simulink model "Final_Minh_Long"  (R2022b)
settings: Solver=VariableStepAuto  StartTime=0.0  StopTime=60  FixedStep=0.001  RelTol=1e-3
undefined symbols (not defined in the file): h, km, m, s, smiData, X, Y, Z
libraries: sm_lib x424, nesl_utility x32, aerolibconvert2 x25, simulink_extras x14, autolibshared x5, simulink x2
(part 1 of 11)
settings Model: Creator=dangm  LastModifiedBy=Lenovo
settings SolverCC: ZeroCrossAlgorithm=Adaptive  AlgebraicLoopSolver=LineSearch
settings DebuggingCC: IgnoredZcDiagnostic=none  UnconnectedInputMsg=warning  UnconnectedOutputMsg=warning  UnconnectedLineMsg=warning  SFMachineParentedDataDiag=warning
settings ModelReferenceCC: EnableRefExpFcnMdlSchedulingChecks=on

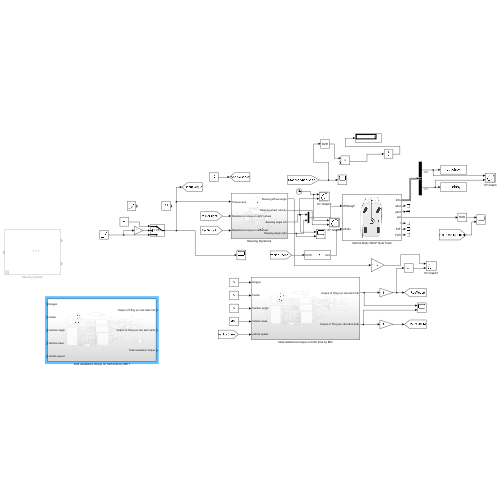
[thumbnail: Simulink's stored preview of the top-level diagram]
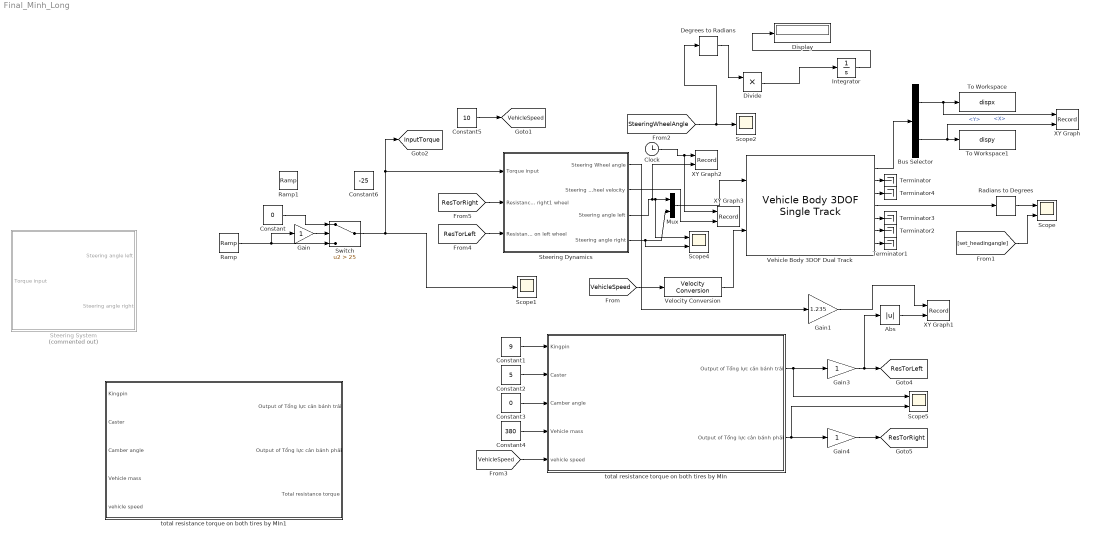
== system Final_Minh_Long ==
  Abs : Abs  SaturateOnIntegerOverflow=off
  Bus Selector : BusSelector  OutputSignals=InertFrm.Cg.Disp.X,InertFrm.Cg.Disp.Y
  Clock : Clock
  Constant : Constant  Value=0
  Constant1 : Constant  Value=9
  Constant2 : Constant  Value=5
  Constant3 : Constant  Value=0
  Constant4 : Constant  Value=380
  Constant5 : Constant  Value=10
  Constant6 : Constant  Value=-25
  Degrees to Radians : simulink_extras/Transformations/Degrees to Radians
  Display : Display
  Divide : Product  Inputs=**
  Gain : Gain
  Gain1 : Gain  Gain=1.235
  Gain3 : Gain
  Gain4 : Gain
  Integrator : Integrator
  Mux : Mux  Inputs=2
  Radians to Degrees : simulink_extras/Transformations/Radians to Degrees
  Ramp : simulink/Sources/Ramp  slope=1  start=0  InitialOutput=0
  Ramp1 : simulink/Sources/Ramp  slope=0.01  start=0  InitialOutput=0
  Scope : Scope  NumInputPorts=2
  Scope1 : Scope
  Scope2 : Scope
  Scope4 : Scope  NumInputPorts=2
  Scope5 : Scope  NumInputPorts=2
  Steering Dynamics : Subsystem
  Steering System : Subsystem  Commented=on
      mask Display: image('D:\MATLAB Projects\MATLAB_EPS_Complete_09_05\CapsoneProject\duy\mask\power-steering-2255498-1882000.png'); % Use "Edit Image" on toolstrip to change.
  Switch : Switch  Criteria=u2 > Threshold  Threshold=25  SaturateOnIntegerOverflow=off  InputSameDT=off
  Terminator{,1..4} (5 alike) : Terminator
  To Workspace : ToWorkspace  VariableName=dispx  SaveFormat=Structure With Time  SampleTime=-1
  To Workspace1 : ToWorkspace  VariableName=dispy  SaveFormat=Structure With Time  SampleTime=-1
  Vehicle Body 3DOF Dual Track : autolibshared/Vehicle Body 3DOF Single Track  trackMode=Dual  inputMode=External longitudinal velocity  frontSteerMode=on  rearSteerMode=off  windMode=off  muMode=off  extFMode=off  extMMode=off  htchFMode=off  htchMMode=off  extXo=off  extpsio=off  extxdoto=off  extro=off  extYo=off  extTamb=off  extydoto=off  aMode=2  NF=2  NR=2  m=1520  a=1.4  b=1.4  h=0.35  dh=1  hh=0.2  X_o=0  xdot_o=0  CalphaMode=off  sigmaMode=on  d=0  hl=0  w=[1.4,1.4]  Cy_f=12e3  Cy_r=11e3  sigma_f=.1  sigma_r=.1  alpha_f_brk=[-.1 .1]  Cy_f_data=[-9e3 9e3]  alpha_r_brk=[-.1 .1]  Cy_r_data=[-9e3 9e3]  Y_o=0  ydot_o=0  Izz=4000  psi_o=0  r_o=0  Af=2  Cd=.3  Cl=.1  Cpm=.1  beta_w=[0:0.01:0.3]  Cs=[0:0.03:0.9]  Cym=[0:0.01:0.3]  Pabs=101325  Tair=273  g=9.81  mu=1  xdot_tol=.01  Fznom=5000  Fxtire_sat=7e4  Fytire_sat=7e4  longOff=0  latOff=0  vertOff=0  wrapAng=off
  Velocity Conversion : aerolibconvert2/Velocity Conversion  IU=km/h  OU=m/s
  XY Graph : Record  FileSettingsInternal="{\"entries\":[{\"content\":{\"excelSettings\":{\"content\":{},\"type\":\"Streamout.ExcelSettings\"}},\"type\":\"Streamout.FileSettingStorage\",\"uuid\":\"20573330-48e2-4ccb-9357-96704c9ba468\"}],\"packageUris\":[\"http://schema.mathworks.com/mf0/streamout_blocks/R2020a\"],\"version\":\"1.0\"}"  Layout=[1 1]  SignalsInternal="{\"entries\":[{\"content\":{\"signals\":[{\"content\":{\"blockPath\":[\"Final_Minh_Long/XY Graph\"],\"channel\":[],\"dimensions\":[1],\"domain\":\"Final_Minh_Long/XY Graph\",\"lineColor\":\"#a2142f\",\"plots\":[1],\"port\":1,\"sid\":[\"\"],\"signalID\":3944,\"signalName\":\"<X>\"},\"type\":\"RecordBlkView.Signal\",\"uuid\":\"90b13e37-3913-4415-9f79-a5536db0b110\"},{\"content\":{\"blockPath\":[\"Final_Minh_Long/XY Graph\"],\"channel\":[],\"dimensions\":[1],\"domain\":\"Final_Minh_Long/XY Graph\",\"lineColor\":\"#139fff\",\"plots\":[1],\"port\":2,\"sid\":[\"\"],\"signalID\":3948,\"signalName\":\"<Y>\"},\"type\":\"RecordBlkView.Signal\",\"uuid\":\"8d3dad9d-9c13-4f6a-a484-58929b97bed7\"}]},\"type\":\"RecordBlkView.InputSignals\",\"uuid\":\"2abae3c5-8f03-4ddf-bdef-c417156e70b2\"}],\"packageUris\":[\"http://schema.mathworks.com/mf0/streamout_blocks/R2020a\"],\"version\":\"1.0\"}"  VisualizationBindings="{\"xyplotplugin\":{\"info\":[{\"series\":[{\"bindingParametersList\":[{\"parameter\":\"X-Axis\",\"signalID\":3944,\"signalName\":\"<X>\"},{\"parameter\":\"Y-Axis\",\"signalID\":3948,\"signalName\":\"<Y>\"}],\"seriesID\":57916}],\"subplotID\":1}]}}"  CompatibilityTag=XY  st=-1
  XY Graph1 : Record  FileSettingsInternal="{\"entries\":[{\"content\":{\"excelSettings\":{\"content\":{},\"type\":\"Streamout.ExcelSettings\"}},\"type\":\"Streamout.FileSettingStorage\",\"uuid\":\"0a007d86-071d-43f5-8a56-b751ea0b846e\"}],\"packageUris\":[\"http://schema.mathworks.com/mf0/streamout_blocks/R2020a\"],\"version\":\"1.0\"}"  Layout=[1 1]  SignalsInternal="{\"entries\":[{\"content\":{\"signals\":[{\"content\":{\"blockPath\":[\"Final_Minh_Long/XY Graph1\"],\"channel\":[],\"dimensions\":[1],\"domain\":\"Final_Minh_Long/XY Graph1\",\"lineColor\":\"#a2142f\",\"plots\":[1],\"port\":1,\"sid\":[\"\"],\"signalID\":3952,\"signalName\":\"Gain1\"},\"type\":\"RecordBlkView.Signal\",\"uuid\":\"8b19a18e-6e3d-497a-a0a3-2aad5dbcfb8c\"},{\"content\":{\"blockPath\":[\"Final_Minh_Long/XY Graph1\"],\"channel\":[],\"dimensions\":[1],\"domain\":\"Final_Minh_Long/XY Graph1\",\"lineColor\":\"#139fff\",\"plots\":[1],\"port\":2,\"sid\":[\"\"],\"signalID\":3956,\"signalName\":\"Abs\"},\"type\":\"RecordBlkView.Signal\",\"uuid\":\"0fb60146-9920-4be2-b459-6142f6fc3ce0\"}]},\"type\":\"RecordBlkView.InputSignals\",\"uuid\":\"4d27a010-d85b-49c4-9162-294f8bc1f08d\"}],\"packageUris\":[\"http://schema.mathworks.com/mf0/streamout_blocks/R2020a\"],\"version\":\"1.0\"}"  VisualizationBindings="{\"xyplotplugin\":{\"info\":[{\"series\":[{\"bindingParametersList\":[{\"parameter\":\"X-Axis\",\"signalID\":3952,\"signalName\":\"Gain1\"},{\"parameter\":\"Y-Axis\",\"signalID\":3956,\"signalName\":\"Abs\"}],\"seriesID\":31774}],\"subplotID\":1}]}}"  CompatibilityTag=XY  st=-1
  XY Graph2 : Record  FileSettingsInternal="{\"entries\":[{\"content\":{\"excelSettings\":{\"content\":{},\"type\":\"Streamout.ExcelSettings\"}},\"type\":\"Streamout.FileSettingStorage\",\"uuid\":\"818af3ad-4e78-4077-87d8-8a147781513b\"}],\"packageUris\":[\"http://schema.mathworks.com/mf0/streamout_blocks/R2020a\"],\"version\":\"1.0\"}"  Layout=[1 1]  SignalsInternal="{\"entries\":[{\"content\":{\"signals\":[{\"content\":{\"blockPath\":[\"Final_Minh_Long/XY Graph2\"],\"channel\":[],\"dimensions\":[1],\"domain\":\"Final_Minh_Long/XY Graph2\",\"lineColor\":\"#a2142f\",\"plots\":[1],\"port\":1,\"sid\":[\"\"],\"signalID\":3960,\"signalName\":\"Clock\"},\"type\":\"RecordBlkView.Signal\",\"uuid\":\"f2a8c6ab-ef34-4918-a704-d61b8c315ada\"},{\"content\":{\"blockPath\":[\"Final_Minh_Long/XY Graph2\"],\"channel\":[],\"dimensions\":[1],\"domain\":\"Final_Minh_Long/XY Graph2\",\"lineColor\":\"#139fff\",\"plots\":[1],\"port\":2,\"sid\":[\"\"],\"signalID\":3964,\"signalName\":\"Steering Dynamics:3\"},\"type\":\"RecordBlkView.Signal\",\"uuid\":\"651528bd-dcb0-49c9-af94-924e8d19c524\"}]},\"type\":\"RecordBlkView.InputSignals\",\"uuid\":\"f8b33b09-6380-4f4b-ae2b-7c84b78898a2\"}],\"packageUris\":[\"http://schema.mathworks.com/mf0/streamout_blocks/R2020a\"],\"version\":\"1.0\"}"  VisualizationBindings="{\"xyplotplugin\":{\"info\":[{\"series\":[{\"bindingParametersList\":[{\"parameter\":\"X-Axis\",\"signalID\":3960,\"signalName\":\"Clock\"},{\"parameter\":\"Y-Axis\",\"signalID\":3964,\"signalName\":\"Steering Dynamics:3\"}],\"seriesID\":31371}],\"subplotID\":1}]}}"  CompatibilityTag=XY  st=-1
  XY Graph3 : Record  FileSettingsInternal="{\"entries\":[{\"content\":{\"excelSettings\":{\"content\":{},\"type\":\"Streamout.ExcelSettings\"}},\"type\":\"Streamout.FileSettingStorage\",\"uuid\":\"88566568-d1b9-45b3-b9ae-773698c52360\"}],\"packageUris\":[\"http://schema.mathworks.com/mf0/streamout_blocks/R2020a\"],\"version\":\"1.0\"}"  Layout=[1 1]  SignalsInternal="{\"entries\":[{\"content\":{\"signals\":[{\"content\":{\"blockPath\":[\"Final_Minh_Long/XY Graph3\"],\"channel\":[],\"dimensions\":[1],\"domain\":\"Final_Minh_Long/XY Graph3\",\"lineColor\":\"#a2142f\",\"plots\":[1],\"port\":1,\"sid\":[\"\"],\"signalID\":3968,\"signalName\":\"Clock\"},\"type\":\"RecordBlkView.Signal\",\"uuid\":\"cc2650eb-84e2-4086-96a6-97ce3e4d41ed\"},{\"content\":{\"blockPath\":[\"Final_Minh_Long/XY Graph3\"],\"channel\":[],\"dimensions\":[1],\"domain\":\"Final_Minh_Long/XY Graph3\",\"lineColor\":\"#139fff\",\"plots\":[1],\"port\":2,\"sid\":[\"\"],\"signalID\":3972,\"signalName\":\"Steering Dynamics:2\"},\"type\":\"RecordBlkView.Signal\",\"uuid\":\"bed2728c-8836-43cf-9a2f-cf65613dc0e0\"}]},\"type\":\"RecordBlkView.InputSignals\",\"uuid\":\"f26de753-25e0-4fe3-9a2b-f6db05d15f66\"}],\"packageUris\":[\"http://schema.mathworks.com/mf0/streamout_blocks/R2020a\"],\"version\":\"1.0\"}"  VisualizationBindings="{\"xyplotplugin\":{\"info\":[{\"series\":[{\"bindingParametersList\":[{\"parameter\":\"X-Axis\",\"signalID\":3968,\"signalName\":\"Clock\"},{\"parameter\":\"Y-Axis\",\"signalID\":3972,\"signalName\":\"Steering Dynamics:2\"}],\"seriesID\":17655}],\"subplotID\":1}]}}"  CompatibilityTag=XY  st=-1
  total resistance torque on both tires by MIn : Subsystem
  total resistance torque on both tires by MIn1 : Subsystem
  tag scope: InputTorque=global, ResTorLeft=global, ResTorRight=global, VehicleSpeed=global
  wires:
  Mux/1 -> Vehicle Body 3DOF Dual Track/1
  Vehicle Body 3DOF Dual Track/7 -> Terminator1/1
  Vehicle Body 3DOF Dual Track/6 -> Terminator2/1
  Vehicle Body 3DOF Dual Track/5 -> Terminator3/1
  Vehicle Body 3DOF Dual Track/1 -> Bus Selector/1
  Bus Selector/1 -> XY Graph/1, To Workspace/1  "<X>"
  Bus Selector/2 -> XY Graph/2, To Workspace1/1  "<Y>"
  Velocity Conversion/1 -> Vehicle Body 3DOF Dual Track/2
  [VehicleSpeed] -> Velocity Conversion/1
  Constant5/1 -> [VehicleSpeed]
  Vehicle Body 3DOF Dual Track/2 -> Terminator/1
  Vehicle Body 3DOF Dual Track/3 -> Terminator4/1
  Vehicle Body 3DOF Dual Track/4 -> Radians to Degrees/1
  Radians to Degrees/1 -> Scope/1
  [set_headingangle] -> Scope/2
  [SteeringWheelAngle] -> Scope2/1, Degrees to Radians/1
  Gain4/1 -> [ResTorRight]
  Gain3/1 -> Abs/1, [ResTorLeft]
  Constant1/1 -> total resistance torque on both tires by MIn/1(Kingpin)
  Constant4/1 -> total resistance torque on both tires by MIn/4(Vehicle mass)
  Constant3/1 -> total resistance torque on both tires by MIn/3(Camber angle)
  Constant2/1 -> total resistance torque on both tires by MIn/2(Caster)
  total resistance torque on both tires by MIn/1(Output of Tổng lực cản bánh trái) -> Scope5/1, Gain3/1
  total resistance torque on both tires by MIn/2(Output of Tổng lực cản bánh phải) -> Gain4/1, Scope5/2
  [VehicleSpeed] -> total resistance torque on both tires by MIn/5("vehicle speed ")
  Degrees to Radians/1 -> Divide/1
  Divide/1 -> Integrator/1
  Integrator/1 -> Display/1
  Constant/1 -> Switch/1
  Switch/1 -> Scope1/1, [InputTorque], Steering Dynamics/1(Torque input)
  Ramp/1 -> Gain/1, Switch/3
  Steering Dynamics/3(Steering angle left) -> XY Graph2/2, Scope4/1, Mux/1
  Steering Dynamics/4(Steering angle right) -> Scope4/2, Mux/2
  [ResTorRight] -> Steering Dynamics/2(Resistance torque on right1 wheel)
  [ResTorLeft] -> Steering Dynamics/3(Resistance torque on left wheel)
  Steering Dynamics/1(Steering Wheel angle) -> Gain1/1
  Gain/1 -> Switch/2
  Abs/1 -> XY Graph1/2
  Gain1/1 -> XY Graph1/1
  Clock/1 -> XY Graph3/1, XY Graph2/1
  Steering Dynamics/2(Steering wheel velocity) -> XY Graph3/2

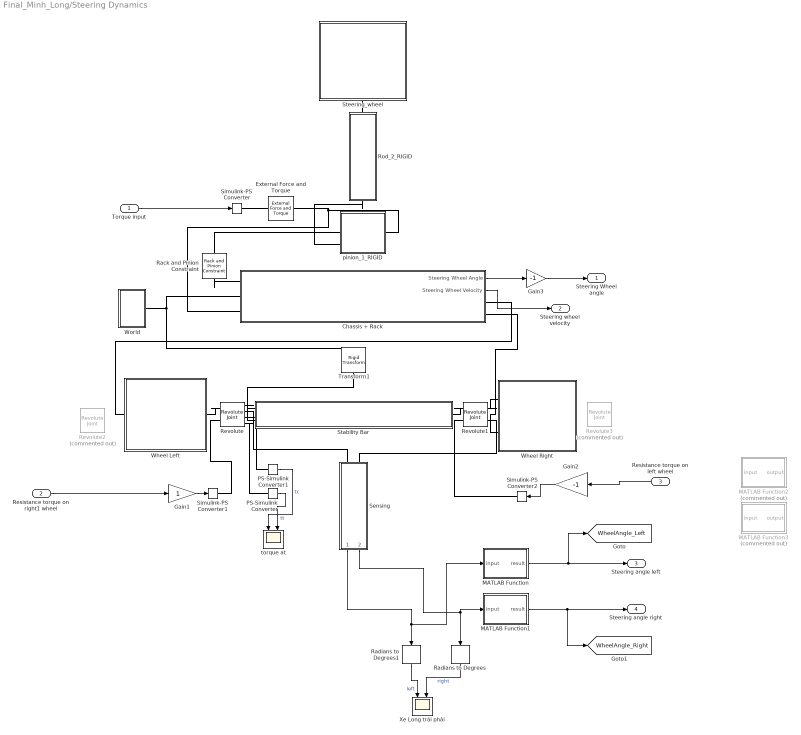
== system Final_Minh_Long/Steering Dynamics ==
  Torque input : Inport
  Resistance torque on right1 wheel : Inport  Port=2
  Resistance torque on left wheel : Inport  Port=3
  Chassis + Rack : Subsystem
      mask Display: image('$imagefile'); % Use "Edit Image" on toolstrip to change.
  External Force and Torque : sm_lib/Forces and Torques/External Force and Torque  ForceResolutionFrame=AttachedFrame  EnableForceX=off  EnableForceY=off  EnableForceZ=off  EnableForce=off  TorqueResolutionFrame=AttachedFrame  EnableTorqueX=off  EnableTorqueY=off  EnableTorqueZ=on  EnableTorque=off
  Gain1 : Gain
  Gain2 : Gain  Gain=-1
  Gain3 : Gain  Gain=-1
  MATLAB Function : MATLAB Function  TreatAsAtomicUnit=on
  MATLAB Function1 : MATLAB Function  TreatAsAtomicUnit=on
  MATLAB Function2 : MATLAB Function  Commented=on  TreatAsAtomicUnit=on
  MATLAB Function3 : MATLAB Function  Commented=on  TreatAsAtomicUnit=on
  PS-Simulink Converter : nesl_utility/PS-Simulink Converter  PhysicalDomain=network_engine_domain  SubClassName=ps_output  LeftPortType=input  RightPortType=output  PseudoPeriodic=off  Frequencies=[]  VectorFormat=1-D array  Unit=inherit  AffineConversion=off
  PS-Simulink Converter1 : nesl_utility/PS-Simulink Converter  PhysicalDomain=network_engine_domain  SubClassName=ps_output  LeftPortType=input  RightPortType=output  PseudoPeriodic=off  Frequencies=[]  VectorFormat=1-D array  Unit=inherit  AffineConversion=off
  Rack and Pinion Constraint : sm_lib/Gears and Couplings/Gears/Rack and Pinion Constraint  PinionRadius=30  PinionRadiusUnits=mm
  Radians to Degrees : simulink_extras/Transformations/Radians to Degrees
  Radians to Degrees1 : simulink_extras/Transformations/Radians to Degrees
  Revolute : sm_lib/Joints/Revolute Joint  JointMode=Normal  SenseConstraintForce=off  SenseConstraintForceX=off  SenseConstraintForceY=off  SenseConstraintForceZ=off  SenseConstraintTorque=on  SenseConstraintTorqueX=off  SenseConstraintTorqueY=off  SenseConstraintTorqueZ=off  SenseTotalForce=off  SenseTotalForceX=off  SenseTotalForceY=off  SenseTotalForceZ=off  SenseTotalTorque=on  SenseTotalTorqueX=off  SenseTotalTorqueY=off  SenseTotalTorqueZ=off  CompositeWrenchDir=BaseOnFollower  CompositeWrenchFrame=FollowerFrame  EquilibriumPosition=0  EquilibriumPositionUnits=deg  SpringStiffness=0.0524-0.0524  SpringStiffnessUnits=N*m/deg  DampingCoefficient=1.5-1.5+0.1  DampingCoefficientUnits=N*m/(deg/s)  TorqueActuationMode=InputTorque  MotionActuationMode=ComputedMotion  SensePosition=on  SenseVelocity=off  SenseAcceleration=off  SenseTorqueForce=off  SenseLowerLimitTorqueForce=off  SenseUpperLimitTorqueForce=off  LowerLimitSpecify=on  LowerLimitBound=-89.68-28.95  LowerLimitBoundUnits=deg  LowerLimitStiffness=1e4  LowerLimitStiffnessUnits=N*m/deg  LowerLimitDamping=100  LowerLimitDampingUnits=N*m/(deg/s)  LowerLimitTransitionRegionWidth=0.1  LowerLimitTransitionRegionWidthUnits=deg  UpperLimitSpecify=on  UpperLimitBound=-89.68+18.80  UpperLimitBoundUnits=deg  UpperLimitStiffness=1e4  UpperLimitStiffnessUnits=N*m/deg  UpperLimitDamping=100  UpperLimitDampingUnits=N*m/(deg/s)  UpperLimitTransitionRegionWidth=0.1  UpperLimitTransitionRegionWidthUnits=deg  PositionTargetSpecify=on  PositionTargetPriority=High  PositionTargetValue=-89.678329494  PositionTargetValueUnits=deg  VelocityTargetSpecify=on  VelocityTargetPriority=High  VelocityTargetValue=0  VelocityTargetValueUnits=deg/s
  Revolute1 : sm_lib/Joints/Revolute Joint  JointMode=Normal  SenseConstraintForce=off  SenseConstraintForceX=off  SenseConstraintForceY=off  SenseConstraintForceZ=off  SenseConstraintTorque=off  SenseConstraintTorqueX=off  SenseConstraintTorqueY=off  SenseConstraintTorqueZ=off  SenseTotalForce=off  SenseTotalForceX=off  SenseTotalForceY=off  SenseTotalForceZ=off  SenseTotalTorque=off  SenseTotalTorqueX=off  SenseTotalTorqueY=off  SenseTotalTorqueZ=off  CompositeWrenchDir=FollowerOnBase  CompositeWrenchFrame=FollowerFrame  EquilibriumPosition=0  EquilibriumPositionUnits=deg  SpringStiffness=0  SpringStiffnessUnits=N*m/deg  DampingCoefficient=0.1  DampingCoefficientUnits=N*m/(deg/s)  TorqueActuationMode=InputTorque  MotionActuationMode=ComputedMotion  SensePosition=on  SenseVelocity=off  SenseAcceleration=off  SenseTorqueForce=off  SenseLowerLimitTorqueForce=off  SenseUpperLimitTorqueForce=off  LowerLimitSpecify=on  LowerLimitBound=-89.68-28.95  LowerLimitBoundUnits=deg  LowerLimitStiffness=1e4  LowerLimitStiffnessUnits=N*m/deg  LowerLimitDamping=100  LowerLimitDampingUnits=N*m/(deg/s)  LowerLimitTransitionRegionWidth=0.1  LowerLimitTransitionRegionWidthUnits=deg  UpperLimitSpecify=on  UpperLimitBound=-89.68+18.80  UpperLimitBoundUnits=deg  UpperLimitStiffness=1e4  UpperLimitStiffnessUnits=N*m/deg  UpperLimitDamping=100  UpperLimitDampingUnits=N*m/(deg/s)  UpperLimitTransitionRegionWidth=0.1  UpperLimitTransitionRegionWidthUnits=deg  PositionTargetSpecify=on  PositionTargetPriority=Low  PositionTargetValue=smiData.RevoluteJoint(2).Rz.Pos-2.7  PositionTargetValueUnits=deg  VelocityTargetSpecify=on  VelocityTargetPriority=High  VelocityTargetValue=0  VelocityTargetValueUnits=deg/s
  Revolute2 : sm_lib/Joints/Revolute Joint  Commented=on  JointMode=Normal  SenseConstraintForce=off  SenseConstraintForceX=off  SenseConstraintForceY=off  SenseConstraintForceZ=off  SenseConstraintTorque=off  SenseConstraintTorqueX=off  SenseConstraintTorqueY=off  SenseConstraintTorqueZ=off  SenseTotalForce=off  SenseTotalForceX=off  SenseTotalForceY=off  SenseTotalForceZ=off  SenseTotalTorque=off  SenseTotalTorqueX=off  SenseTotalTorqueY=off  SenseTotalTorqueZ=off  CompositeWrenchDir=BaseOnFollower  CompositeWrenchFrame=FollowerFrame  EquilibriumPosition=0  EquilibriumPositionUnits=deg  SpringStiffness=0.0524-0.0524+0.1  SpringStiffnessUnits=N*m/deg  DampingCoefficient=1.5-1.5+0.1  DampingCoefficientUnits=N*m/(deg/s)  TorqueActuationMode=InputTorque  MotionActuationMode=ComputedMotion  SensePosition=on  SenseVelocity=off  SenseAcceleration=off  SenseTorqueForce=off  SenseLowerLimitTorqueForce=off  SenseUpperLimitTorqueForce=off  LowerLimitSpecify=on  LowerLimitBound=-2+0.089+0.071  LowerLimitBoundUnits=rad  LowerLimitStiffness=1e4  LowerLimitStiffnessUnits=N*m/deg  LowerLimitDamping=100  LowerLimitDampingUnits=N*m/(deg/s)  LowerLimitTransitionRegionWidth=0.1  LowerLimitTransitionRegionWidthUnits=deg  UpperLimitSpecify=on  UpperLimitBound=-1-0.195-0.106  UpperLimitBoundUnits=rad  UpperLimitStiffness=1e4  UpperLimitStiffnessUnits=N*m/deg  UpperLimitDamping=100  UpperLimitDampingUnits=N*m/(deg/s)  UpperLimitTransitionRegionWidth=0.1  UpperLimitTransitionRegionWidthUnits=deg  PositionTargetSpecify=on  PositionTargetPriority=High  PositionTargetValue=-89.678329494  PositionTargetValueUnits=deg  VelocityTargetSpecify=on  VelocityTargetPriority=High  VelocityTargetValue=0  VelocityTargetValueUnits=deg/s
  Revolute3 : sm_lib/Joints/Revolute Joint  Commented=on  JointMode=Normal  SenseConstraintForce=off  SenseConstraintForceX=off  SenseConstraintForceY=off  SenseConstraintForceZ=off  SenseConstraintTorque=off  SenseConstraintTorqueX=off  SenseConstraintTorqueY=off  SenseConstraintTorqueZ=off  SenseTotalForce=off  SenseTotalForceX=off  SenseTotalForceY=off  SenseTotalForceZ=off  SenseTotalTorque=off  SenseTotalTorqueX=off  SenseTotalTorqueY=off  SenseTotalTorqueZ=off  CompositeWrenchDir=FollowerOnBase  CompositeWrenchFrame=FollowerFrame  EquilibriumPosition=0  EquilibriumPositionUnits=deg  SpringStiffness=0.1  SpringStiffnessUnits=N*m/deg  DampingCoefficient=0.1  DampingCoefficientUnits=N*m/(deg/s)  TorqueActuationMode=InputTorque  MotionActuationMode=ComputedMotion  SensePosition=on  SenseVelocity=off  SenseAcceleration=off  SenseTorqueForce=off  SenseLowerLimitTorqueForce=off  SenseUpperLimitTorqueForce=off  LowerLimitSpecify=off  LowerLimitBound=-2  LowerLimitBoundUnits=rad  LowerLimitStiffness=1e4  LowerLimitStiffnessUnits=N*m/deg  LowerLimitDamping=100  LowerLimitDampingUnits=N*m/(deg/s)  LowerLimitTransitionRegionWidth=0.1  LowerLimitTransitionRegionWidthUnits=deg  UpperLimitSpecify=off  UpperLimitBound=-1  UpperLimitBoundUnits=rad  UpperLimitStiffness=1e4  UpperLimitStiffnessUnits=N*m/deg  UpperLimitDamping=100  UpperLimitDampingUnits=N*m/(deg/s)  UpperLimitTransitionRegionWidth=0.1  UpperLimitTransitionRegionWidthUnits=deg  PositionTargetSpecify=on  PositionTargetPriority=Low  PositionTargetValue=smiData.RevoluteJoint(2).Rz.Pos-2.7  PositionTargetValueUnits=deg  VelocityTargetSpecify=on  VelocityTargetPriority=High  VelocityTargetValue=0  VelocityTargetValueUnits=deg/s
  Rod_2_RIGID : Subsystem
      mask Display: image('rod.png'); % Use "Edit Image" on toolstrip to change.
  "Sensing " : Subsystem
  Simulink-PS Converter : nesl_utility/Simulink-PS Converter  PhysicalDomain=network_engine_domain  SubClassName=ps_input  LeftPortType=input  RightPortType=output  PseudoPeriodic=off  Frequencies=[]  NoiseDistribution=none  NoiseParameters=[]  Unit=N*m  AffineConversion=off  FilteringAndDerivatives=provide  SimscapeFilterOrder=1  InputFilterTimeConstant=0.001  UdotUserProvided=0
  Simulink-PS Converter1 : nesl_utility/Simulink-PS Converter  PhysicalDomain=network_engine_domain  SubClassName=ps_input  LeftPortType=input  RightPortType=output  PseudoPeriodic=off  Frequencies=[]  NoiseDistribution=none  NoiseParameters=[]  Unit=N*m  AffineConversion=off  FilteringAndDerivatives=provide  SimscapeFilterOrder=1  InputFilterTimeConstant=0.001  UdotUserProvided=0
  Simulink-PS Converter2 : nesl_utility/Simulink-PS Converter  PhysicalDomain=network_engine_domain  SubClassName=ps_input  LeftPortType=input  RightPortType=output  PseudoPeriodic=off  Frequencies=[]  NoiseDistribution=none  NoiseParameters=[]  Unit=N*m  AffineConversion=off  FilteringAndDerivatives=provide  SimscapeFilterOrder=2  InputFilterTimeConstant=0.001  UdotUserProvided=0
  Stability Bar : Subsystem
      mask Display: image('$imagefile'); % Use "Edit Image" on toolstrip to change.
  Steering_wheel : Subsystem
      mask Display: image('$imagefile'); % Use "Edit Image" on toolstrip to change.
  Transform1 : sm_lib/Frames and Transforms/Rigid Transform  TranslationMethod=Cartesian  TranslationStandardOffset=0  TranslationLengthUnit=mm  TranslationStandardAxis=+Z  TranslationCartesianOffset=smiData.RigidTransform(48).translation  TranslationROffset=0  TranslationROffsetUnits=m  TranslationZOffset=0  TranslationZOffsetUnits=m  TranslationThetaOffset=0  TranslationThetaOffsetUnits=deg  RotationMethod=ArbitraryAxis  RotationAngleUnits=rad  RotationStandardAxis=+Z  RotationAngle=smiData.RigidTransform(48).angle  RotationArbitraryAxis=smiData.RigidTransform(48).axis  FollAlignAxisA=+X  BaseAlignAxisA=+Y  FollAlignAxisB=+Y  BaseAlignAxisB=+Z  RotationSequenceAxes=FollowerAxes  RotationSequence=XYX  RotationSequenceAngles=[0 0 0]  RotationSequenceAnglesUnits=deg  RotationMatrix=[1 0 0; 0 1 0; 0 0 1]  Quaternion=[1 0 0 0]
  Wheel Left : Subsystem
      mask Display: image('$imagefile'); % Use "Edit Image" on toolstrip to change.
  Wheel Right : Subsystem
      mask Display: image('$imagefile'); % Use "Edit Image" on toolstrip to change.
  World : Subsystem
  Xe Long trái phải : Scope  NumInputPorts=2
  pinion_1_RIGID : Subsystem
      mask Display: image('pinion.png'); % Use "Edit Image" on toolstrip to change.
  "torque at " : Scope  NumInputPorts=2
  Steering Wheel angle : Outport
  Steering wheel velocity : Outport  Port=2
  Steering angle left : Outport  Port=3
  Steering angle right : Outport  Port=4
  tag scope: WheelAngle_Left=global, WheelAngle_Right=global
  wires:
  "Sensing "/2(Steering angle right (rad)) -> MATLAB Function1/1(input), Radians to Degrees/1
  Radians to Degrees/1 -> Xe Long trái phải/2  "right"
  Radians to Degrees1/1 -> Xe Long trái phải/1  "left"
  Chassis + Rack/2(Steering Wheel Velocity) -> Steering wheel velocity/1
  Chassis + Rack/1(Steering Wheel Angle) -> Gain3/1
  Resistance torque on right1 wheel/1 -> Gain1/1
  Resistance torque on left wheel/1 -> Gain2/1
  Gain1/1 -> Simulink-PS Converter1/1
  Gain2/1 -> Simulink-PS Converter2/1
  MATLAB Function/1(result) -> [WheelAngle_Left], Steering angle left/1
  MATLAB Function1/1(result) -> [WheelAngle_Right], Steering angle right/1
  "Sensing "/1(Steering angle left (rad)) -> Radians to Degrees1/1, MATLAB Function/1(input)
  PS-Simulink Converter1/1 -> "torque at "/1  "tc"
  PS-Simulink Converter/1 -> "torque at "/2  "tt"
  Torque input/1 -> Simulink-PS Converter/1
  Gain3/1 -> Steering Wheel angle/1
  connections:
  Revolute/RConn2 -- "Sensing "/LConn1
  Simulink-PS Converter/RConn1 -- External Force and Torque/LConn1
  Chassis + Rack/LConn2 -- World/LConn1 -- Transform1/LConn1
  Rack and Pinion Constraint/RConn1 -- Chassis + Rack/LConn1
  Revolute1/RConn2 -- "Sensing "/LConn2
  Rack and Pinion Constraint/LConn1 -- pinion_1_RIGID/LConn2
  Transform1/RConn1 -- Stability Bar/LConn2
  Chassis + Rack/LConn3 -- pinion_1_RIGID/RConn1 -- External Force and Torque/RConn1
  Chassis + Rack/RConn1 -- Wheel Left/LConn1
  Revolute1/RConn1 -- Wheel Right/LConn1
  Chassis + Rack/RConn2 -- Wheel Right/LConn2
  Revolute1/LConn1 -- Stability Bar/RConn1
  Revolute/RConn1 -- Stability Bar/LConn1
  Revolute/LConn1 -- Wheel Left/RConn1
  Rod_2_RIGID/RConn1 -- pinion_1_RIGID/LConn3
  Steering_wheel/LConn1 -- Rod_2_RIGID/LConn1
  Simulink-PS Converter1/RConn1 -- Revolute/LConn2
  Revolute1/LConn2 -- Simulink-PS Converter2/RConn1
  Revolute/RConn3 -- PS-Simulink Converter1/LConn1
  Revolute/RConn4 -- PS-Simulink Converter/LConn1

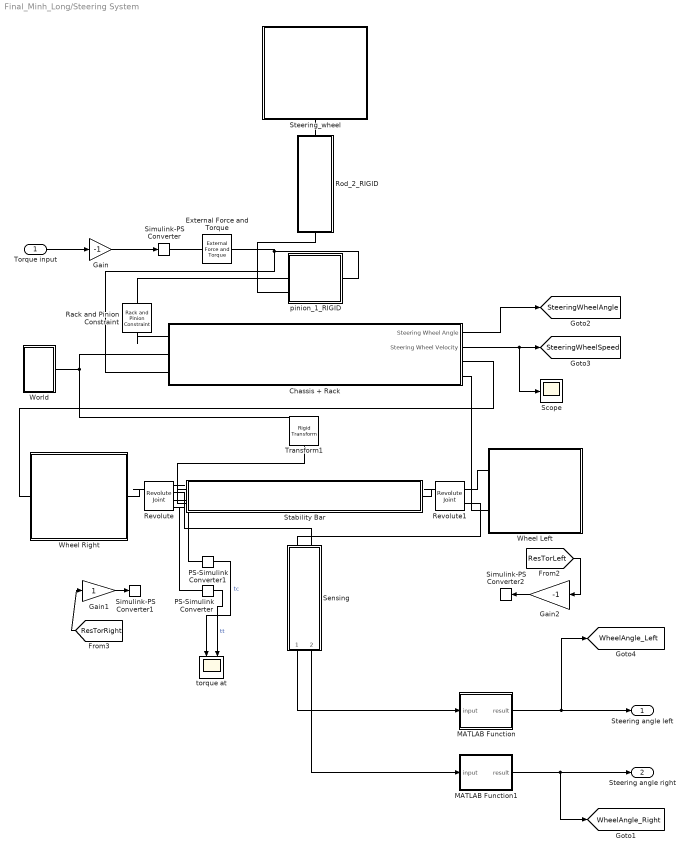
== system Final_Minh_Long/Steering System ==
  Torque input : Inport
  Chassis + Rack : Subsystem
      mask Display: image('$imagefile'); % Use "Edit Image" on toolstrip to change.
  External Force and Torque : sm_lib/Forces and Torques/External Force and Torque  ForceResolutionFrame=AttachedFrame  EnableForceX=off  EnableForceY=off  EnableForceZ=off  EnableForce=off  TorqueResolutionFrame=AttachedFrame  EnableTorqueX=off  EnableTorqueY=off  EnableTorqueZ=on  EnableTorque=off
  Gain : Gain  Gain=-1
  Gain1 : Gain
  Gain2 : Gain  Gain=-1
  MATLAB Function : MATLAB Function  TreatAsAtomicUnit=on
  MATLAB Function1 : MATLAB Function  TreatAsAtomicUnit=on
  PS-Simulink Converter : nesl_utility/PS-Simulink Converter  PhysicalDomain=network_engine_domain  SubClassName=ps_output  LeftPortType=input  RightPortType=output  PseudoPeriodic=off  Frequencies=[]  VectorFormat=1-D array  Unit=inherit  AffineConversion=off
  PS-Simulink Converter1 : nesl_utility/PS-Simulink Converter  PhysicalDomain=network_engine_domain  SubClassName=ps_output  LeftPortType=input  RightPortType=output  PseudoPeriodic=off  Frequencies=[]  VectorFormat=1-D array  Unit=inherit  AffineConversion=off
  Rack and Pinion Constraint : sm_lib/Gears and Couplings/Gears/Rack and Pinion Constraint  PinionRadius=30  PinionRadiusUnits=mm
  Revolute : sm_lib/Joints/Revolute Joint  JointMode=Normal  SenseConstraintForce=off  SenseConstraintForceX=off  SenseConstraintForceY=off  SenseConstraintForceZ=off  SenseConstraintTorque=on  SenseConstraintTorqueX=off  SenseConstraintTorqueY=off  SenseConstraintTorqueZ=off  SenseTotalForce=off  SenseTotalForceX=off  SenseTotalForceY=off  SenseTotalForceZ=off  SenseTotalTorque=on  SenseTotalTorqueX=off  SenseTotalTorqueY=off  SenseTotalTorqueZ=off  CompositeWrenchDir=BaseOnFollower  CompositeWrenchFrame=FollowerFrame  EquilibriumPosition=0  EquilibriumPositionUnits=deg  SpringStiffness=0.0524-0.0524+0.1  SpringStiffnessUnits=N*m/deg  DampingCoefficient=1.5-1.5+0.1  DampingCoefficientUnits=N*m/(deg/s)  TorqueActuationMode=InputTorque  MotionActuationMode=ComputedMotion  SensePosition=on  SenseVelocity=off  SenseAcceleration=off  SenseTorqueForce=off  SenseLowerLimitTorqueForce=off  SenseUpperLimitTorqueForce=off  LowerLimitSpecify=on  LowerLimitBound=-89.68-28.95  LowerLimitBoundUnits=deg  LowerLimitStiffness=1e4  LowerLimitStiffnessUnits=N*m/deg  LowerLimitDamping=100  LowerLimitDampingUnits=N*m/(deg/s)  LowerLimitTransitionRegionWidth=0.1  LowerLimitTransitionRegionWidthUnits=deg  UpperLimitSpecify=on  UpperLimitBound=-89.68+18.80  UpperLimitBoundUnits=deg  UpperLimitStiffness=1e4  UpperLimitStiffnessUnits=N*m/deg  UpperLimitDamping=100  UpperLimitDampingUnits=N*m/(deg/s)  UpperLimitTransitionRegionWidth=0.1  UpperLimitTransitionRegionWidthUnits=deg  PositionTargetSpecify=on  PositionTargetPriority=High  PositionTargetValue=-89.678329494  PositionTargetValueUnits=deg  VelocityTargetSpecify=on  VelocityTargetPriority=High  VelocityTargetValue=0  VelocityTargetValueUnits=deg/s
  Revolute1 : sm_lib/Joints/Revolute Joint  JointMode=Normal  SenseConstraintForce=off  SenseConstraintForceX=off  SenseConstraintForceY=off  SenseConstraintForceZ=off  SenseConstraintTorque=off  SenseConstraintTorqueX=off  SenseConstraintTorqueY=off  SenseConstraintTorqueZ=off  SenseTotalForce=off  SenseTotalForceX=off  SenseTotalForceY=off  SenseTotalForceZ=off  SenseTotalTorque=off  SenseTotalTorqueX=off  SenseTotalTorqueY=off  SenseTotalTorqueZ=off  CompositeWrenchDir=FollowerOnBase  CompositeWrenchFrame=FollowerFrame  EquilibriumPosition=0  EquilibriumPositionUnits=deg  SpringStiffness=0.1  SpringStiffnessUnits=N*m/deg  DampingCoefficient=0.1  DampingCoefficientUnits=N*m/(deg/s)  TorqueActuationMode=InputTorque  MotionActuationMode=ComputedMotion  SensePosition=on  SenseVelocity=off  SenseAcceleration=off  SenseTorqueForce=off  SenseLowerLimitTorqueForce=off  SenseUpperLimitTorqueForce=off  LowerLimitSpecify=on  LowerLimitBound=-89.68-28.95  LowerLimitBoundUnits=deg  LowerLimitStiffness=1e4  LowerLimitStiffnessUnits=N*m/deg  LowerLimitDamping=100  LowerLimitDampingUnits=N*m/(deg/s)  LowerLimitTransitionRegionWidth=0.1  LowerLimitTransitionRegionWidthUnits=deg  UpperLimitSpecify=on  UpperLimitBound=-89.68+18.80  UpperLimitBoundUnits=deg  UpperLimitStiffness=1e4  UpperLimitStiffnessUnits=N*m/deg  UpperLimitDamping=100  UpperLimitDampingUnits=N*m/(deg/s)  UpperLimitTransitionRegionWidth=0.1  UpperLimitTransitionRegionWidthUnits=deg  PositionTargetSpecify=on  PositionTargetPriority=Low  PositionTargetValue=smiData.RevoluteJoint(2).Rz.Pos-2.7  PositionTargetValueUnits=deg  VelocityTargetSpecify=on  VelocityTargetPriority=High  VelocityTargetValue=0  VelocityTargetValueUnits=deg/s
  Rod_2_RIGID : Subsystem
      mask Display: image('rod.png'); % Use "Edit Image" on toolstrip to change.
  Scope : Scope
  "Sensing " : Subsystem
  Simulink-PS Converter : nesl_utility/Simulink-PS Converter  PhysicalDomain=network_engine_domain  SubClassName=ps_input  LeftPortType=input  RightPortType=output  PseudoPeriodic=off  Frequencies=[]  NoiseDistribution=none  NoiseParameters=[]  Unit=N*m  AffineConversion=off  FilteringAndDerivatives=provide  SimscapeFilterOrder=1  InputFilterTimeConstant=0.001  UdotUserProvided=0
  Simulink-PS Converter1 : nesl_utility/Simulink-PS Converter  PhysicalDomain=network_engine_domain  SubClassName=ps_input  LeftPortType=input  RightPortType=output  PseudoPeriodic=off  Frequencies=[]  NoiseDistribution=none  NoiseParameters=[]  Unit=N*m  AffineConversion=off  FilteringAndDerivatives=provide  SimscapeFilterOrder=1  InputFilterTimeConstant=0.001  UdotUserProvided=0
  Simulink-PS Converter2 : nesl_utility/Simulink-PS Converter  PhysicalDomain=network_engine_domain  SubClassName=ps_input  LeftPortType=input  RightPortType=output  PseudoPeriodic=off  Frequencies=[]  NoiseDistribution=none  NoiseParameters=[]  Unit=N*m  AffineConversion=off  FilteringAndDerivatives=provide  SimscapeFilterOrder=2  InputFilterTimeConstant=0.001  UdotUserProvided=0
  Stability Bar : Subsystem
      mask Display: image('$imagefile'); % Use "Edit Image" on toolstrip to change.
  Steering_wheel : Subsystem
      mask Display: image('$imagefile'); % Use "Edit Image" on toolstrip to change.
  Transform1 : sm_lib/Frames and Transforms/Rigid Transform  TranslationMethod=Cartesian  TranslationStandardOffset=0  TranslationLengthUnit=mm  TranslationStandardAxis=+Z  TranslationCartesianOffset=smiData.RigidTransform(48).translation  TranslationROffset=0  TranslationROffsetUnits=m  TranslationZOffset=0  TranslationZOffsetUnits=m  TranslationThetaOffset=0  TranslationThetaOffsetUnits=deg  RotationMethod=ArbitraryAxis  RotationAngleUnits=rad  RotationStandardAxis=+Z  RotationAngle=smiData.RigidTransform(48).angle  RotationArbitraryAxis=smiData.RigidTransform(48).axis  FollAlignAxisA=+X  BaseAlignAxisA=+Y  FollAlignAxisB=+Y  BaseAlignAxisB=+Z  RotationSequenceAxes=FollowerAxes  RotationSequence=XYX  RotationSequenceAngles=[0 0 0]  RotationSequenceAnglesUnits=deg  RotationMatrix=[1 0 0; 0 1 0; 0 0 1]  Quaternion=[1 0 0 0]
  Wheel Left : Subsystem
      mask Display: image('$imagefile'); % Use "Edit Image" on toolstrip to change.
  Wheel Right : Subsystem
      mask Display: image('$imagefile'); % Use "Edit Image" on toolstrip to change.
  World : Subsystem
  pinion_1_RIGID : Subsystem
  "torque at " : Scope  NumInputPorts=2
  Steering angle left : Outport
  Steering angle right : Outport  Port=2
  tag scope: SteeringWheelAngle=global, SteeringWheelSpeed=global, WheelAngle_Left=global, WheelAngle_Right=global
  wires:
  "Sensing "/2(Steering angle right (rad)) -> MATLAB Function1/1(input)
  Chassis + Rack/2(Steering Wheel Velocity) -> Scope/1, [SteeringWheelSpeed]
  Chassis + Rack/1(Steering Wheel Angle) -> [SteeringWheelAngle]
  [ResTorRight] -> Gain1/1
  [ResTorLeft] -> Gain2/1
  Gain1/1 -> Simulink-PS Converter1/1
  Gain2/1 -> Simulink-PS Converter2/1
  MATLAB Function/1(result) -> [WheelAngle_Left], Steering angle left/1
  MATLAB Function1/1(result) -> [WheelAngle_Right], Steering angle right/1
  Torque input/1 -> Gain/1
  "Sensing "/1(Steering angle left (rad)) -> MATLAB Function/1(input)
  PS-Simulink Converter1/1 -> "torque at "/1  "tc"
  PS-Simulink Converter/1 -> "torque at "/2  "tt"
  Gain/1 -> Simulink-PS Converter/1
  connections:
  Revolute/RConn2 -- "Sensing "/LConn2
  Simulink-PS Converter/RConn1 -- External Force and Torque/LConn1
  Chassis + Rack/LConn2 -- World/LConn1 -- Transform1/LConn1
  Rack and Pinion Constraint/RConn1 -- Chassis + Rack/LConn1
  Revolute1/RConn2 -- "Sensing "/LConn1
  Rack and Pinion Constraint/LConn1 -- pinion_1_RIGID/LConn2
  Transform1/RConn1 -- Stability Bar/LConn2
  Chassis + Rack/LConn3 -- pinion_1_RIGID/RConn1 -- External Force and Torque/RConn1
  Chassis + Rack/RConn1 -- Wheel Right/LConn1
  Revolute1/RConn1 -- Wheel Left/LConn1
  Chassis + Rack/RConn2 -- Wheel Left/LConn2
  Revolute1/LConn1 -- Stability Bar/RConn1
  Revolute/RConn1 -- Stability Bar/LConn1
  Revolute/LConn1 -- Wheel Right/RConn1
  Rod_2_RIGID/RConn1 -- pinion_1_RIGID/LConn3
  Steering_wheel/LConn1 -- Rod_2_RIGID/LConn1
  Revolute/RConn3 -- PS-Simulink Converter1/LConn1
  Revolute/RConn4 -- PS-Simulink Converter/LConn1

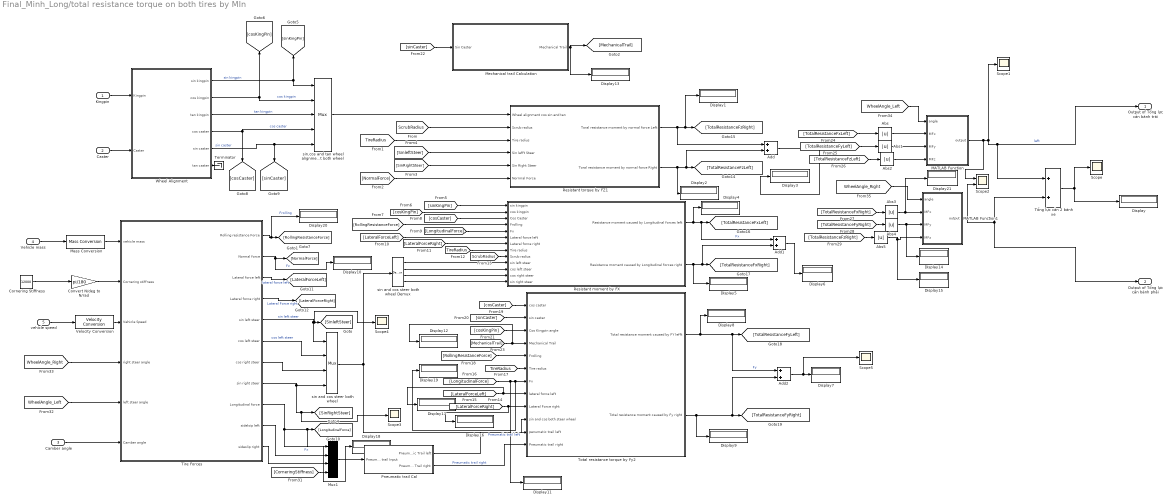
== system Final_Minh_Long/total resistance torque on both tires by MIn ==
  Kingpin : Inport
  Caster : Inport  Port=2
  Camber angle : Inport  Port=3
  Vehicle mass : Inport  Port=4
  "vehicle speed " : Inport  Port=5
  Abs{,1..5} (6 alike) : Abs  SaturateOnIntegerOverflow=off
  Add : Sum
  Add1 : Sum
  Add2 : Sum
  Convert N/deg to N/rad : Gain  Gain=pi/180
  Cornering Stiffness : Constant  Value=12000
  Display{,1..21} (22 alike) : Display
  MATLAB Function : MATLAB Function  TreatAsAtomicUnit=on
  MATLAB Function1 : MATLAB Function  TreatAsAtomicUnit=on
  Mass Conversion : aerolibconvert2/Mass Conversion  IU=kg  OU=kg
  "Mechanical trail Calculation " : Subsystem
  Mux1 : Mux
  Pneumatic trail Cal : Subsystem
  Resistant moment by FX : Subsystem
  Resistant torque by FZ1 : Subsystem
  Scope{,1,3..5} (5 alike) : Scope
  Scope2 : Scope  NumInputPorts=2
  Terminator : Terminator
  Tire Forces : Subsystem
  Total resistance torque by Fy2 : Subsystem
  Tổng lực cản 2 bánh xe : Sum
  Velocity Conversion : aerolibconvert2/Velocity Conversion  IU=km/h  OU=m/s
  Wheel Alignment : Subsystem
  sin and cos steer both wheel : Mux
  sin and cos steer both wheel Demux : Demux
  sin,cos and tan wheel alignment both wheel : Mux  Inputs=5
  Output of Tổng lực cản bánh trái : Outport
  Output of Tổng lực cản bánh phải : Outport  Port=2
  wires:
  Kingpin/1 -> Wheel Alignment/1(Kingpin)
  Wheel Alignment/6(tan caster) -> Terminator/1
  Vehicle mass/1 -> Mass Conversion/1
  Mass Conversion/1 -> Tire Forces/1(vehicle mass)
  Cornering Stiffness/1 -> Convert N/deg to N/rad/1
  Caster/1 -> Wheel Alignment/2(Caster)
  "vehicle speed "/1 -> Velocity Conversion/1
  [WheelAngle_Right] -> Tire Forces/4("right steer angle ")
  [WheelAngle_Left] -> Tire Forces/5("left steer angle ")
  Velocity Conversion/1 -> Tire Forces/3(Vehicle Speed)
  Tire Forces/11(sideslip right) -> Mux1/3
  Tire Forces/10(sidelsip left) -> Mux1/2
  Tire Forces/9(Longitudinal force) -> Mux1/1, Display18/1, [LongitudinalForce]  "Fx"
  Mux1/1 -> Pneumatic trail Cal/1(Pneumatic trail Input)
  Pneumatic trail Cal/2(Pneumatic Trail right) -> Total resistance torque by Fy2/12(Pneumatic trail right)  "Pneumatic trail right"
  Pneumatic trail Cal/1(Pneumatic Trail left) -> Total resistance torque by Fy2/11(penumatic trail left)  "Pneumatic trail left"
  Tire Forces/5(sin left steer) -> sin and cos steer both wheel/1, Scope4/1, [SinleftSteer]  "sin left steer"
  Tire Forces/6(cos left steer) -> sin and cos steer both wheel/2  "cos left steer"
  Tire Forces/7(cos right steer) -> sin and cos steer both wheel/3
  Tire Forces/8(sin right steer) -> Scope3/1, [SinRightSteer], sin and cos steer both wheel/4
  sin and cos steer both wheel/1 -> Total resistance torque by Fy2/10(sin and cos both steer wheel), sin and cos steer both wheel Demux/1
  Wheel Alignment/1(sin kingpin) -> sin,cos and tan wheel alignment both wheel/1, [sinKingPin]  "sin kingpin"
  Wheel Alignment/2(cos kingpin) -> [cosKingPin], sin,cos and tan wheel alignment both wheel/2  "cos kingpin"
  Wheel Alignment/3(tan kingpin) -> sin,cos and tan wheel alignment both wheel/3  "tan kingpin"
  Wheel Alignment/4(cos caster) -> sin,cos and tan wheel alignment both wheel/4, [cosCaster]  "cos caster"
  Wheel Alignment/5(sin caster) -> [sinCaster], sin,cos and tan wheel alignment both wheel/5  "sin caster"
  sin,cos and tan wheel alignment both wheel/1 -> Resistant torque by FZ1/1("Wheel alignment cos sin and tan ")
  Tire Forces/2(Normal force) -> Display10/1, [NormalForce]  "Fz"
  [ScrubRadius] -> Resistant torque by FZ1/2(Scrub radius)
  [TireRadius] -> Resistant torque by FZ1/3(Tire radius)
  [sinKingPin] -> Resistant moment by FX/1(sin kingpin)
  [cosKingPin] -> Resistant moment by FX/2(cos kingpin)
  Tire Forces/1(Rolling resistance Force) -> Display20/1, [RollingResistanceForce]  "Frolling"
  [RollingResistanceForce] -> Resistant moment by FX/4(Frolling)
  [cosCaster] -> Resistant moment by FX/3(Cos Caster)
  [LongitudinalForce] -> Resistant moment by FX/5(Fx)
  Tire Forces/3(Lateral force left) -> [LateralForceLeft]  "lateral force left"
  Tire Forces/4(Lateral force right) -> [LateralForceRight]  "Lateral Force right"
  [LateralForceLeft] -> Resistant moment by FX/6(Lateral force left)
  [LateralForceRight] -> Resistant moment by FX/7(Lateral force right)
  [TireRadius] -> Resistant moment by FX/8(Tire radius)
  [ScrubRadius] -> Resistant moment by FX/9(Scrub radius)
  [LateralForceRight] -> Display16/1, Total resistance torque by Fy2/9(Lateral Force right)
  [TireRadius] -> Total resistance torque by Fy2/6(Tire radius)
  [RollingResistanceForce] -> Total resistance torque by Fy2/5(Frolling)
  [cosCaster] -> Total resistance torque by Fy2/1(cos caster)
  sin and cos steer both wheel Demux/1 -> Resistant moment by FX/10(sin left steer)
  sin and cos steer both wheel Demux/2 -> Resistant moment by FX/11(cos left steer)
  sin and cos steer both wheel Demux/3 -> Resistant moment by FX/12(cos right steer)
  sin and cos steer both wheel Demux/4 -> Resistant moment by FX/13(sin right steer)
  Resistant moment by FX/1(Resistance moment caused by Longitudinal forces left) -> Display4/1, Add1/1, [TotalResistanceFxLeft]  "Fx"
  Resistant moment by FX/2(Resistance moment caused by Longitudinal forces right) -> Display5/1, Add1/2, [TotalResistanceFxRight]
  Total resistance torque by Fy2/2(Total resistance moment caused by Fy right) -> Display9/1, Add2/2, [TotalResistanceFyRight]
  Total resistance torque by Fy2/1("Total resistance moment caused by FY lefft ") -> Display8/1, Add2/1, [TotalResistanceFyLeft]  "Fy"
  [TotalResistanceFxLeft] -> Abs/1
  [TotalResistanceFyLeft] -> Abs1/1
  [TotalResistanceFzLeft] -> Abs2/1
  [TotalResistanceFxRight] -> Abs3/1
  [TotalResistanceFyRight] -> Abs4/1
  [TotalResistanceFzRight] -> Abs5/1
  Tổng lực cản 2 bánh xe/1 -> Scope/1, Display/1
  Convert N/deg to N/rad/1 -> Tire Forces/2(Cornering stiffness)
  [CorneringStiffness] -> Mux1/4
  [sinCaster] -> Total resistance torque by Fy2/2(sin caster)
  [cosKingPin] -> Total resistance torque by Fy2/3(Cos Kingpin angle)
  [MechanicalTrail] -> Display12/1, Total resistance torque by Fy2/4(Mechanical Trail)
  [LongitudinalForce] -> Display19/1, Total resistance torque by Fy2/7(Fx), Display11/1
  [LateralForceLeft] -> Display17/1, Total resistance torque by Fy2/8(lateral force left)
  [SinleftSteer] -> Resistant torque by FZ1/4(Sin lefft Steer)
  [SinRightSteer] -> Resistant torque by FZ1/5(Sin Right Steer)
  [NormalForce] -> Resistant torque by FZ1/6(Norrmal Force)
  Resistant torque by FZ1/1(Toral resistance moment by normal force Left) -> Add/1, Display1/1, [TotalResistanceFzRight]
  Resistant torque by FZ1/2(Toral resistance moment by normal force Right) -> Display2/1, Add/2, [TotalResistanceFzLeft]
  Add/1 -> Display3/1
  Add1/1 -> Display6/1
  Add2/1 -> Scope5/1, Display7/1
  "Mechanical trail Calculation "/1(Mechanical Trail) -> [MechanicalTrail], Display13/1
  [sinCaster] -> "Mechanical trail Calculation "/1(Sin Caster)
  Camber angle/1 -> Tire Forces/6(Camber angle)
  MATLAB Function/1(output) -> Scope2/1, Output of Tổng lực cản bánh trái/1, Tổng lực cản 2 bánh xe/1, Scope1/1  "left"
  [WheelAngle_Left] -> MATLAB Function/1(angle)
  MATLAB Function1/1(output) -> Scope2/2, Output of Tổng lực cản bánh phải/1, Tổng lực cản 2 bánh xe/2
  [WheelAngle_Right] -> MATLAB Function1/1(angle)
  Abs/1 -> MATLAB Function/2(MFx)
  Abs1/1 -> MATLAB Function/3(MFy)
  Abs2/1 -> MATLAB Function/4(MFz)
  Abs3/1 -> Display21/1, MATLAB Function1/2(MFx)
  Abs4/1 -> Display14/1, MATLAB Function1/3(MFy)
  Abs5/1 -> Display15/1, MATLAB Function1/4(MFz)
